simulink model "A4_11_leadlag"  (Simulink 7.4)
settings: Solver=FixedStepDiscrete  StartTime=0.0  StopTime=10  RelTol=1e-3
values from neighbouring files (symbols this model uses):
  a = sign(diff(data.signals.values(ind_max_first:end,1)))    [A4_10_plotSinusComparison.m]
undefined symbols (not defined in the file or in its folder): alag, dend, Kp, numd, tl, tllag
libraries: DCmotor_library x1
settings Model: Creator=Natalia  LastModifiedBy=ma
settings DebuggingCC: StrictBusMsg=ErrorLevel1
settings HardwareCC: ProdIntDivRoundTo=Zero  ProdEndianess=LittleEndian  ProdHWDeviceType=Generic->32-bit x86 compatible
settings RTWCC: SystemTargetFile=rtwin.tlc  TemplateMakefile=rtwin.tmf  Description=Real-Time Windows Target  ProcessScript=rtwin_make_rtw_hook  RTWCompilerOptimization=On
settings CodeAppCC: MaxIdLength=95  CustomSymbolStrType=$N$R$M_T
settings TargetCC: TargetLibSuffix=_rtwin.lib  TargetPreCompLibLocation=C:\Program Files\MATLAB\R2012b\toolbox\rtw\targets\rtwin\lib\win64  TargetFunctionLibrary=ANSI_C  IsPILTarget=off  MatFileLogging=on  EnableShiftOperators=on
settings CustomProperty: DataType=string  Value=C:/PROGRA~1/MATLAB/R2012b/toolbox/rtw/targets/rtwin

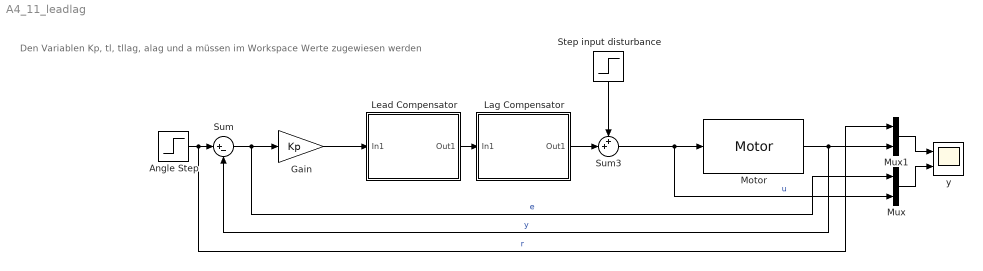
== system A4_11_leadlag ==
  note: Den Variablen
      | Kp, tl, tllag, alag und a
      | müssen im Workspace
      | Werte zugewiesen werden
  Angle Step : Step  After=10  SampleTime=0.01
  Gain : Gain  Gain=Kp
  Lag Compensator : Subsystem  mask(DiscretizedTransferFcn){Numerator=[1 1/tllag], Denominator=[1 1/(tllag*alag)], AbsTol=auto, SampleTime=0.01, method=tustin, Wc=1}
      mask prompts: Numerator "Numerator (enter in s-domain:)"; Denominator "Denominator (enter in s-domain:)"; AbsTol "Absolute tolerance:"; SampleTime "Sample time:"; Wc "Critical Frequency (Hz):"
      mask help: Continuous mask uses c2d to transform parameters onto the Discrete Transfer function block inside.
      mask init:
      | st=SampleTime;
      | if length(st)>1
      |     st=SampleTime(1);
      | end
      | if(st>0)
      |     [numd,dend] = sldiscutil('disctransferfcn',{st,method,Wc,Numerator,Denominator});
      | end	
      | s = get_param(gcb,'maskvalues');
      | nums = s{1};
      | dens = s{2};
      | %numc = eval(nums);
      | %denc = eval(dens);
      | sldiscutil('inittfmask', st);
      | if(st==0)
      | set_param([gcb '/Transfer Fcn'], 'AbsoluteTolerance', AbsTol);
      | end
      mask StyleString: edit,edit,edit,edit,popup(zoh|foh|tustin|prewarp|matched),edit
      mask CallbackString: ||||hidecrit|
      mask Display:
      | dpoly(nums,dens)
      | text( 0.5, 1.0, method, 'verticalAlignment','top')
  Lead Compensator : Subsystem  mask(DiscretizedTransferFcn){Numerator=[tl 1], Denominator=[tl*a 1], AbsTol=auto, SampleTime=0.01, method=tustin, Wc=1}
      mask prompts: Numerator "Numerator (enter in s-domain:)"; Denominator "Denominator (enter in s-domain:)"; AbsTol "Absolute tolerance:"; SampleTime "Sample time:"; Wc "Critical Frequency (Hz):"
      mask help: Continuous mask uses c2d to transform parameters onto the Discrete Transfer function block inside.
      mask init: same as A4_11_leadlag/Lag Compensator
      mask StyleString: edit,edit,edit,edit,popup(zoh|foh|tustin|prewarp|matched),edit
      mask CallbackString: ||||hidecrit|
      mask Display:
      | dpoly(nums,dens)
      | text( 0.5, 1.0, method, 'verticalAlignment','top')
  Motor : DCmotor_library/Motor  motoridinput=8  name_signal=Angle  ts=10
  Mux : Mux  Inputs=2
  Mux1 : Mux  Inputs=2
  Step input disturbance : Step  Time=3  After=0  SampleTime=0
  Sum : Sum  Inputs=|+-
  Sum3 : Sum  Inputs=++|
  y : Scope  NumInputPorts=2
      settings: YMin=-25~-700  YMax=50~1500
  wires:
  Angle Step/1 -> Mux1/1, Sum/1  "r"
  Sum/1 -> Mux/1, Gain/1  "e"
  Lead Compensator/1(Out1) -> Lag Compensator/1(In1)
  Motor/1 -> Sum/2, Mux1/2  "y"
  Gain/1 -> Lead Compensator/1(In1)
  Lag Compensator/1(Out1) -> Sum3/2
  Step input disturbance/1 -> Sum3/1
  Sum3/1 -> Mux/2, Motor/1  "u"
  Mux1/1 -> y/1
  Mux/1 -> y/2

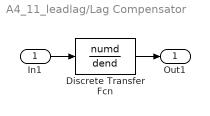
== system A4_11_leadlag/Lag Compensator ==
  In1 : Inport
  Discrete Transfer Fcn : DiscreteTransferFcn  Numerator=numd  Denominator=dend  SampleTime=SampleTime
  Out1 : Outport
  wires:
  In1/1 -> Discrete Transfer Fcn/1
  Discrete Transfer Fcn/1 -> Out1/1

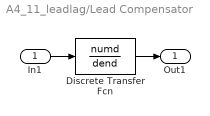
== system A4_11_leadlag/Lead Compensator ==
  In1 : Inport
  Discrete Transfer Fcn : DiscreteTransferFcn  Numerator=numd  Denominator=dend  SampleTime=SampleTime
  Out1 : Outport
  wires:
  Discrete Transfer Fcn/1 -> Out1/1
  In1/1 -> Discrete Transfer Fcn/1
